simulink model "iController"  (R2017b)
settings: Solver=VariableStepAuto  StartTime=0.0  StopTime=10.0  RelTol=1e-3
settings Model: Creator=ohm9xd  LastModifiedBy=ohm9xd

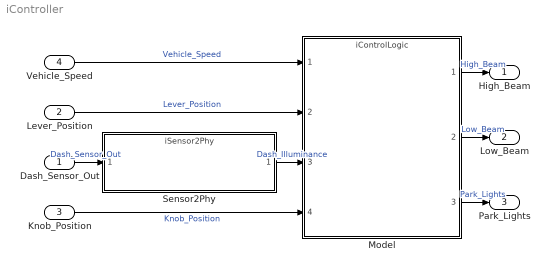
== system iController ==
  Dash_Sensor_Out : Inport
  Lever_Position : Inport  Port=2
  Knob_Position : Inport  Port=3
  Vehicle_Speed : Inport  Port=4
  Model : ModelReference  ModelNameDialog=iControlLogic.slx  SimulationMode=Normal  ModelReferenceVersion=1.4
  Sensor2Phy : ModelReference  ModelNameDialog=iSensor2Phy.slx  SimulationMode=Normal  ModelReferenceVersion=1.1
  High_Beam : Outport
  Low_Beam : Outport  Port=2
  Park_Lights : Outport  Port=3
  wires:
  Sensor2Phy/1 -> Model/3  "Dash_Illuminance"
  Vehicle_Speed/1 -> Model/1  "Vehicle_Speed"
  Knob_Position/1 -> Model/4  "Knob_Position"
  Dash_Sensor_Out/1 -> Sensor2Phy/1  "Dash_Sensor_Out"
  Lever_Position/1 -> Model/2  "Lever_Position"
  Model/1 -> High_Beam/1  "High_Beam"
  Model/2 -> Low_Beam/1  "Low_Beam"
  Model/3 -> Park_Lights/1  "Park_Lights"
